simulink model "HW7_zombies"  (Simulink 7.9)
settings: Solver=ode45  StartTime=0.0  StopTime=6.0  RelTol=1e-3
settings Model: Creator=bazkoale  LastModifiedBy=alex
settings DataIOCC: SignalLoggingSaveFormat=Dataset
settings OptimizationCC: ExpressionDepthLimit=128
settings DebuggingCC: MultiTaskDSMMsg=warning  MultiTaskCondExecSysMsg=none  StrictBusMsg=None
settings RTWCC: IncludeERTFirstTime=on
settings CodeAppCC: CustomSymbolStrType=$N$R$M_T

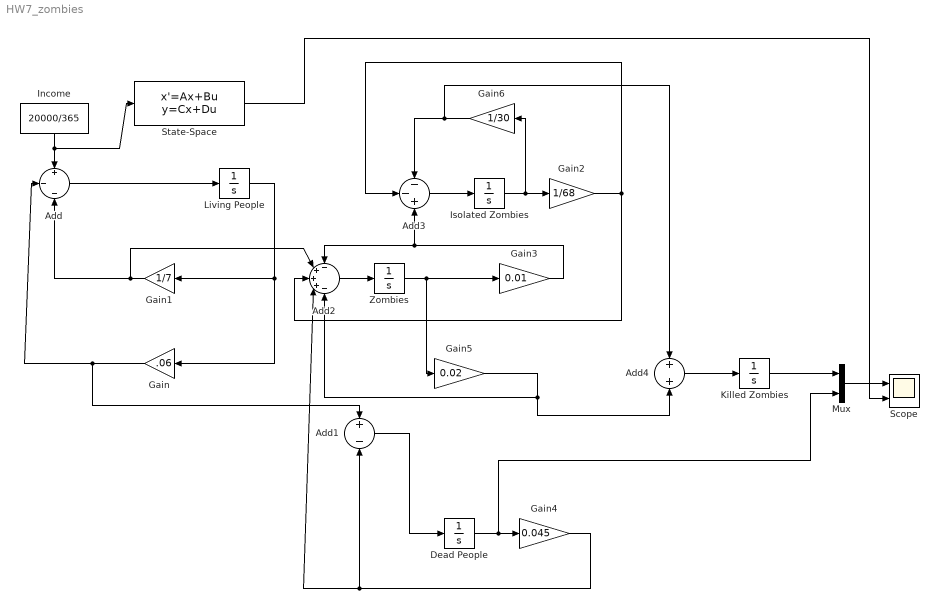
== system HW7_zombies ==
  Add : Sum  Inputs=+|-|-
  Add1 : Sum  Inputs=+-
  Add2 : Sum  Inputs=-+++-
  Add3 : Sum  Inputs=--+
  Add4 : Sum
  "Dead People " : Integrator
  Gain : Gain  Gain=.06
  Gain1 : Gain  Gain=1/7
  Gain2 : Gain  Gain=1/68
  Gain3 : Gain  Gain=0.01
  Gain4 : Gain  Gain=0.045
  Gain5 : Gain  Gain=0.02
  Gain6 : Gain  Gain=1/30
  "Income " : Constant  Value=20000/365
  Isolated Zombies : Integrator
  Killed Zombies : Integrator
  Living People : Integrator  InitialCondition=300000
  Mux : Mux  Inputs=2
  Scope : Scope  NumInputPorts=2
      settings: YMin=-5~-5  YMax=5~5
  State-Space : StateSpace  A=[-1/7-.06 0 0 0 0; .06 -.045 0 0 0; 1/7 .045 -.03 1/68 0; 0 0 .01 -1/68-1/30 0; 0 0 .02 1/30 0]  B=[1; 0; 0; 0; 0]  C=[0 1 0 0 0; 0 0 0 0 1]  D=[0; 0]  X0=[300000; 0; 1; 0; 0]
  Zombies : Integrator
  wires:
  "Income "/1 -> Add/1, State-Space/1
  Add/1 -> Living People/1
  Living People/1 -> Gain1/1, Gain/1
  Gain/1 -> Add1/1, Add/2
  Gain1/1 -> Add2/2, Add/3
  Add1/1 -> "Dead People "/1
  Add2/1 -> Zombies/1
  Isolated Zombies/1 -> Gain6/1, Gain2/1
  Gain2/1 -> Add2/3, Add3/2
  Zombies/1 -> Gain5/1, Gain3/1
  Gain3/1 -> Add2/1, Add3/3
  Add3/1 -> Isolated Zombies/1
  "Dead People "/1 -> Mux/2, Gain4/1
  Gain4/1 -> Add1/2, Add2/4
  Gain5/1 -> Add4/2, Add2/5
  Gain6/1 -> Add4/1, Add3/1
  Add4/1 -> Killed Zombies/1
  Killed Zombies/1 -> Mux/1
  Mux/1 -> Scope/1
  State-Space/1 -> Scope/2
